simulink model "MavicProComplete"  (R2019a)
settings: Solver=VariableStepAuto  StartTime=0  StopTime=125  FixedStep=.01  RelTol=1e-3  EnableMultiTasking=on
InitFcn:
  | load('params/batteryModelSfun.mat');
  | load('params/DJI.mat');
  | load('params/DJIquadModel_X.mat');
  | load('params/motor.mat');
  | load('params/soc_ocv_new.mat');
model workspace (MAT data in the model file):
  MCOS : class17 (value not decoded)
values from neighbouring files (symbols this model uses):
  P = block.ContStates.Data(1)    [quadcopterDynamicsSFunctionMod.m]
  Phi = block.ContStates.Data(4)    [quadcopterDynamicsSFunctionMod.m]
  Psi = block.ContStates.Data(6)    [quadcopterDynamicsSFunctionMod.m]
  Q = block.ContStates.Data(2)    [quadcopterDynamicsSFunctionMod.m]
  R = block.ContStates.Data(3)    [quadcopterDynamicsSFunctionMod.m]
  The = block.ContStates.Data(5)    [quadcopterDynamicsSFunctionMod.m]
  Z = block.ContStates.Data(12)    [quadcopterDynamicsSFunctionMod.m]
undefined symbols (not defined in the file or in its folder): Motor, quadModel
libraries: simulink x7
(part 2 of 2)

== matlab function MavicProComplete/Quadcopter/Powertrain/motorGroup/motor4/motorRotor4/Mechanical part/Propeller model  ==
  data: torque output; rpm input; thrust output
function [torque,thrust] = fcn(rpm)
% angular_velocity in rpm

%coefficient of thrust, empirically derived
coef_t = 2*(10^-15)*rpm^3 - 4*(10^-11)*rpm^2 + 3*(10^-7)*rpm + .1013;
%thrust = coef_t * density of air * velocity^2 * propeller diameter (m) ^4
thrust = coef_t*1.225*(rpm/60)^2*.2^4;
% empirically derived
torque = 4*(10^-14)*rpm^3 +  8*(10^-12)*rpm^2 + 3*(10^-6)*rpm;
end
